simulink model "MontajeFinal"  (R2023a)
settings: Solver=ode4  StartTime=0.0  StopTime=1527  FixedStep=Ts  RelTol=1e-3  EnableMultiTasking=on
PostLoadFcn:
  | Ts=1/200000;L=1.8e-3;w=2*pi*60;C=20e-6;
  | 
  | load('NewCycleFTP75.mat')
  | 
  | Vel=Cycle(:,1);
  | Acc=Cycle(:,2);
InitFcn:
  | Ts=1/200000;L=1.8e-3;w=2*pi*60;C=20e-6;
  | 
  | load('NewCycleFTP75.mat')
  | 
  | Vel=Cycle(:,1);
  | Acc=Cycle(:,2);
values from neighbouring files (symbols this model uses):
  Cycle = [0 0 0 0 0 0 0 0 0 0 0 0 ... (4948 elements, 2474x2)]    [CycleFTP75.mat]    (also in CycleOntibon.mat = [0 0 0 0 0 0 0 0 0 0 0 0 ... (3602 elements, 1801x2)])
undefined symbols (not defined in the file or in its folder): DiscIntNeverNeededParam, sizecont
libraries: simulink x10, spsSeriesRLCBranchLib x8, spsIGBTDiodeLib x6, spsCurrentMeasurementLib x4, spsVoltageMeasurementLib x4, spsGroundLib x4, dspswit3 x2, spsDCVoltageSourceLib x1, spsAsynchronousMachineSIUnitsLib x1, spspowerguiLib x1, slpidlib x1
(part 2 of 2)

== system MontajeFinal/Visualización y Control/SM_Master/Vd_M/Subsystem ==
  X : Inport
  Y : Inport  Port=2
  En : Inport  Port=3
  Divide2 : Product  Inputs=**  OutDataTypeStr=Inherit: Same as first input
  Divide5 : Product  Inputs=**  OutDataTypeStr=Inherit: Same as first input
  X*Y : Outport
  wires:
  X/1 -> Divide2/1
  En/1 -> Divide5/2
  Divide2/1 -> Divide5/1
  Divide5/1 -> X*Y/1
  Y/1 -> Divide2/2

== system MontajeFinal/Visualización y Control/SM_Master/Vd_M/Subsystem1 ==
  X : Inport
  Y : Inport  Port=2
  En : Inport  Port=3
  Divide2 : Product  Inputs=**  OutDataTypeStr=Inherit: Same as first input
  Divide5 : Product  Inputs=**  OutDataTypeStr=Inherit: Same as first input
  X*Y : Outport
  wires:
  X/1 -> Divide2/1
  En/1 -> Divide5/2
  Divide2/1 -> Divide5/1
  Divide5/1 -> X*Y/1
  Y/1 -> Divide2/2

== system MontajeFinal/Visualización y Control/SM_Master/Vd_M1/Subsystem ==
  X : Inport
  Y : Inport  Port=2
  En : Inport  Port=3
  Divide2 : Product  Inputs=**  OutDataTypeStr=Inherit: Same as first input
  Divide5 : Product  Inputs=**  OutDataTypeStr=Inherit: Same as first input
  X*Y : Outport
  wires:
  X/1 -> Divide2/1
  En/1 -> Divide5/2
  Divide2/1 -> Divide5/1
  Divide5/1 -> X*Y/1
  Y/1 -> Divide2/2

== system MontajeFinal/Visualización y Control/SM_Master/Vd_M1/Subsystem1 ==
  X : Inport
  Y : Inport  Port=2
  En : Inport  Port=3
  Divide2 : Product  Inputs=**  OutDataTypeStr=Inherit: Same as first input
  Divide5 : Product  Inputs=**  OutDataTypeStr=Inherit: Same as first input
  X*Y : Outport
  wires:
  X/1 -> Divide2/1
  En/1 -> Divide5/2
  Divide2/1 -> Divide5/1
  Divide5/1 -> X*Y/1
  Y/1 -> Divide2/2

== system MontajeFinal/Visualización y Control/SM_Master/abc//dq_VM/Subsystem2 ==
  alfa : Inport
  beta : Inport  Port=2
  wt : Inport  Port=3
  Fcn : Fcn  Expr=u(1)*cos(u(3))+u(2)*sin(u(3))
  Fcn1 : Fcn  Expr=-u(1)*sin(u(3))+u(2)*cos(u(3))
  Mux : Mux  Inputs=3
  Mux1 : Mux  Inputs=3
  d : Outport
  Q : Outport  Port=2
  wires:
  Fcn/1 -> d/1
  Fcn1/1 -> Q/1
  Mux/1 -> Fcn/1
  alfa/1 -> Mux1/1, Mux/1
  Mux1/1 -> Fcn1/1
  beta/1 -> Mux1/2, Mux/2
  wt/1 -> Mux1/3, Mux/3

== system MontajeFinal/Visualización y Control/SM_Master/abc//dq_VM/abc//alfabeta2 ==
  abc : Inport
  Fcn : Fcn  Expr=1*u(1)-0.5*u(2)-0.5*u(3)
  Fcn1 : Fcn  Expr=0*u(1)+(sqrt(3)/2)*u(2)-(sqrt(3)/2)*u(3)
  Gain : Gain  Gain=k
  alfa : Outport
  Beta : Outport  Port=2
  wires:
  Fcn1/1 -> Beta/1
  Fcn/1 -> alfa/1
  abc/1 -> Gain/1
  Gain/1 -> Fcn/1, Fcn1/1

== system MontajeFinal/Visualización y Control/SM_Master/abc//dq_VM1/Subsystem2 ==
  alfa : Inport
  beta : Inport  Port=2
  wt : Inport  Port=3
  Fcn : Fcn  Expr=u(1)*cos(u(3))+u(2)*sin(u(3))
  Fcn1 : Fcn  Expr=-u(1)*sin(u(3))+u(2)*cos(u(3))
  Mux : Mux  Inputs=3
  Mux1 : Mux  Inputs=3
  d : Outport
  Q : Outport  Port=2
  wires:
  wt/1 -> Mux/3, Mux1/3
  beta/1 -> Mux/2, Mux1/2
  Mux1/1 -> Fcn1/1
  alfa/1 -> Mux/1, Mux1/1
  Mux/1 -> Fcn/1
  Fcn1/1 -> Q/1
  Fcn/1 -> d/1

== system MontajeFinal/Visualización y Control/SM_Master/abc//dq_VM1/abc//alfabeta2 ==
  abc : Inport
  Fcn : Fcn  Expr=1*u(1)-0.5*u(2)-0.5*u(3)
  Fcn1 : Fcn  Expr=0*u(1)+(sqrt(3)/2)*u(2)-(sqrt(3)/2)*u(3)
  Gain : Gain  Gain=k
  alfa : Outport
  Beta : Outport  Port=2
  wires:
  Gain/1 -> Fcn1/1, Fcn/1
  abc/1 -> Gain/1
  Fcn/1 -> alfa/1
  Fcn1/1 -> Beta/1

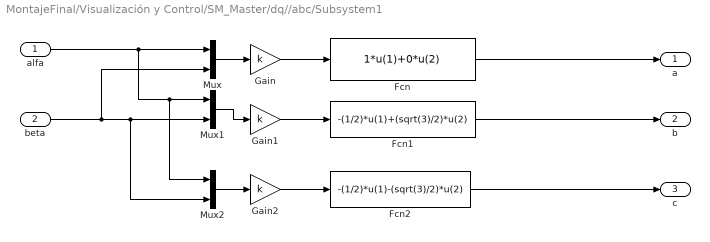
== system MontajeFinal/Visualización y Control/SM_Master/dq//abc/Subsystem1 ==
  alfa : Inport
  beta : Inport  Port=2
  Fcn : Fcn  Expr=1*u(1)+0*u(2)
  Fcn1 : Fcn  Expr=-(1/2)*u(1)+(sqrt(3)/2)*u(2)
  Fcn2 : Fcn  Expr=-(1/2)*u(1)-(sqrt(3)/2)*u(2)
  Gain : Gain  Gain=k
  Gain1 : Gain  Gain=k
  Gain2 : Gain  Gain=k
  Mux : Mux  Inputs=2
  Mux1 : Mux  Inputs=2
  Mux2 : Mux  Inputs=2
  a : Outport
  b : Outport  Port=2
  c : Outport  Port=3
  wires:
  alfa/1 -> Mux2/1, Mux1/1, Mux/1
  Fcn2/1 -> c/1
  beta/1 -> Mux/2, Mux2/2, Mux1/2
  Gain1/1 -> Fcn1/1
  Gain2/1 -> Fcn2/1
  Fcn/1 -> a/1
  Mux/1 -> Gain/1
  Gain/1 -> Fcn/1
  Mux1/1 -> Gain1/1
  Mux2/1 -> Gain2/1
  Fcn1/1 -> b/1

== system MontajeFinal/Visualización y Control/SM_Master/dq//abc/dq//alfabeta1 ==
  d : Inport
  q : Inport  Port=2
  wt : Inport  Port=3
  Fcn2 : Fcn  Expr=u(1)*cos(u(3))-u(2)*sin(u(3))
  Fcn3 : Fcn  Expr=u(1)*sin(u(3))+u(2)*cos(u(3))
  Mux : Mux  Inputs=3
  Mux1 : Mux  Inputs=3
  alfa : Outport
  beta : Outport  Port=2
  wires:
  Fcn3/1 -> beta/1
  wt/1 -> Mux1/3, Mux/3
  q/1 -> Mux1/2, Mux/2
  Mux/1 -> Fcn2/1
  Fcn2/1 -> alfa/1
  d/1 -> Mux1/1, Mux/1
  Mux1/1 -> Fcn3/1

== system MontajeFinal/Visualización y Control/SM_Master/to pwm_M/Salida PWM ==
  "ciclo util " : Inport
  Bus Selector3 : BusSelector  OutputSignals=signal1,signal2,signal3
  Compare To Constant : simulink/Logic and Bit Operations/Compare To Constant  relop=>=  const=0.5  OutDataTypeStr=boolean
  Compare To Constant1 : simulink/Logic and Bit Operations/Compare To Constant  relop=<=  const=0.5  OutDataTypeStr=boolean
  Compare To Constant2 : simulink/Logic and Bit Operations/Compare To Constant  relop=>=  const=0.5  OutDataTypeStr=boolean
  Compare To Constant3 : simulink/Logic and Bit Operations/Compare To Constant  relop=<=  const=0.5  OutDataTypeStr=boolean
  Compare To Constant4 : simulink/Logic and Bit Operations/Compare To Constant  relop=>=  const=0.5  OutDataTypeStr=boolean
  Compare To Constant5 : simulink/Logic and Bit Operations/Compare To Constant  relop=<=  const=0.5  OutDataTypeStr=boolean
  tag scope: p1=global, p2=global, p3=global, p4=global, p5=global, p6=global
  wires:
  "ciclo util "/1 -> Bus Selector3/1
  Bus Selector3/1 -> Compare To Constant1/1, Compare To Constant/1  "<signal1>"
  Bus Selector3/2 -> Compare To Constant2/1, Compare To Constant3/1  "<signal2>"
  Bus Selector3/3 -> Compare To Constant5/1, Compare To Constant4/1  "<signal3>"
  Compare To Constant5/1 -> [p2]
  Compare To Constant4/1 -> [p5]
  Compare To Constant3/1 -> [p6]
  Compare To Constant2/1 -> [p3]
  Compare To Constant1/1 -> [p4]
  Compare To Constant/1 -> [p1]

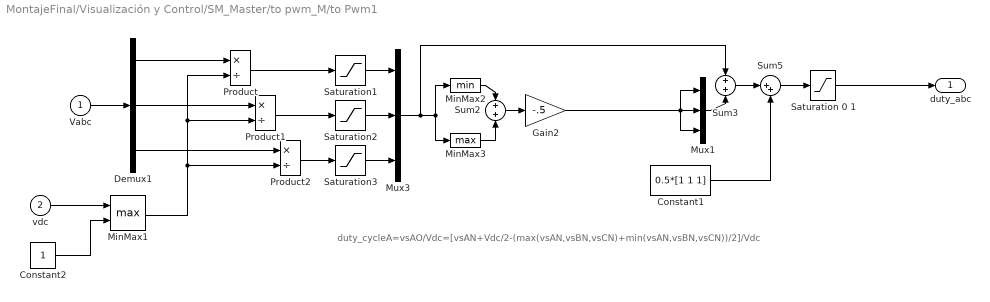
== system MontajeFinal/Visualización y Control/SM_Master/to pwm_M/to Pwm1 ==
  note: duty_cycleA=vsAO/Vdc=[vsAN+Vdc/2-(max(vsAN,vsBN,vsCN)+min(vsAN,vsBN,vsCN))/2]/Vdc
  Vabc : Inport
  vdc : Inport  Port=2
  Constant1 : Constant  Value=0.5*[1 1 1]
  Constant2 : Constant
  Demux1 : Demux  Outputs=3
  Gain2 : Gain  Gain=-.5  SaturateOnIntegerOverflow=on  OutDataTypeStr=Inherit: Same as input  ParamDataTypeStr=Inherit: Same as input
  MinMax1 : MinMax  Function=max  Inputs=2  InputSameDT=on  SaturateOnIntegerOverflow=on
  MinMax2 : MinMax  InputSameDT=on  SaturateOnIntegerOverflow=on
  MinMax3 : MinMax  Function=max  InputSameDT=on  SaturateOnIntegerOverflow=on
  Mux1 : Mux  Inputs=3
  Mux3 : Mux  Inputs=3
  Product : Product  Inputs=*/  SaturateOnIntegerOverflow=on  OutDataTypeStr=Inherit: Same as first input
  Product1 : Product  Inputs=*/  SaturateOnIntegerOverflow=on  OutDataTypeStr=Inherit: Same as first input
  Product2 : Product  Inputs=*/  SaturateOnIntegerOverflow=on  OutDataTypeStr=Inherit: Same as first input
  Saturation 0 1 : Saturate  UpperLimit=0.98  LowerLimit=0.02
  Saturation1 : Saturate  UpperLimit=1/sqrt(3)  LowerLimit=-1/sqrt(3)
  Saturation2 : Saturate  UpperLimit=1/sqrt(3)  LowerLimit=-1/sqrt(3)
  Saturation3 : Saturate  UpperLimit=1/sqrt(3)  LowerLimit=-1/sqrt(3)
  Sum2 : Sum  InputSameDT=on  SaturateOnIntegerOverflow=on  OutDataTypeStr=Inherit: Same as first input
  Sum3 : Sum  InputSameDT=on  SaturateOnIntegerOverflow=on  OutDataTypeStr=Inherit: Same as first input
  Sum5 : Sum  Inputs=|++  InputSameDT=on  SaturateOnIntegerOverflow=on  OutDataTypeStr=Inherit: Same as first input
  duty_abc : Outport
  wires:
  Constant2/1 -> MinMax1/2
  MinMax1/1 -> Product/2, Product1/2, Product2/2
  vdc/1 -> MinMax1/1
  Mux1/1 -> Sum3/2
  Vabc/1 -> Demux1/1
  Saturation 0 1/1 -> duty_abc/1
  Product2/1 -> Saturation3/1
  Demux1/2 -> Product1/1
  Product1/1 -> Saturation2/1
  Product/1 -> Saturation1/1
  Saturation3/1 -> Mux3/3
  Saturation2/1 -> Mux3/2
  Saturation1/1 -> Mux3/1
  Demux1/1 -> Product/1
  Demux1/3 -> Product2/1
  Constant1/1 -> Sum5/2
  Sum3/1 -> Sum5/1
  Gain2/1 -> Mux1/1, Mux1/3, Mux1/2
  Sum2/1 -> Gain2/1
  MinMax2/1 -> Sum2/1
  MinMax3/1 -> Sum2/2
  Mux3/1 -> Sum3/1, MinMax2/1, MinMax3/1
  Sum5/1 -> Saturation 0 1/1
